simulink library "adrc"  (R2021a)
settings: Solver=VariableStepAuto  StartTime=0.0  StopTime=10.0  RelTol=1e-3
settings Model: Creator=onqi  LastModifiedBy=root

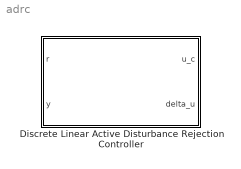
== system adrc ==
  Discrete Linear Active Disturbance Rejection Controller : Subsystem  Variant=on  VariantControl=Choice  mask(Linear Active Disturbance Rejection Control){order=1, b0=1, w_cl=1, k_eso=1, eso_init=[0;0], m_lim=[-inf, inf], r_lim=[-inf, inf], halfgain_ctrl=off, halfgain_obsv=off, inc_form=on, SampleTime=-1}
      mask prompts: order "First- or second-order ADRC"; b0 "Gain parameter b0"; w_cl "Desired closed-loop bandwidth w_cl [rad/s]"; k_eso "Relational observer bandwidth k_eso"; eso_init "Initial state of extended state observer"; m_lim "Magnitude limit of controller [lo, hi]"; r_lim "Rate limit of controller [lo, hi]"; halfgain_ctrl "Toggle half-gain tuning for controller"; halfgain_obsv "Toggle half-gain tuning for observer"; inc_form "Incremental form of ADRC"; SampleTime "Simulink:blkprm_prompts:AllBlksSampleTime"
      mask help:
      | Linear Active Disturbance Rejection Control block implementing the algorithms described in
      |
      | - Practical Active Disturbance Rejection Control: Bumpless Transfer, Rate Limitation and Incremental Algorithm, Gernot Herbst
      | - Half-Gain Tuning for Active Disturbance Rejection Control, Herbst et al.
      mask init:
      | ADRC_INC_FORM = inc_form;
      | 
      | if order == 1
      |     Ad = [[1, SampleTime];[0, 1]];
      |     Bd = [b0 * SampleTime; 0];
      |     Cd = [1, 0];
      |     Dd = 0;
      |     % Controller parameters for closed-loop dynamics
      |     t_settle = 4 / w_cl;
      |     sCL = -4 / t_settle;
      |     Kp = -2 * sCL;
      |     % Observer dynamics
      |     sESO = k_eso * sCL;
      |     zESO = exp(sESO * SampleTime);
      | 
      |     % Observer gains resulting in common-location observer poles
      |     L = [1 - zESO^2; (1 / SampleTime) * (1 - zESO)^2];
      | 
      |     % Controller gains
      |     w = [Kp / b0; 1 / b0];
      | 
      | elseif order == 2
      |     Ad = [[1, SampleTime, (SampleTime^2) / 2]; [0, 1, SampleTime]; [0, 0, 1]];
      |     Bd = [b0 * (SampleTime^2) / 2; b0 * SampleTime; 0];
      |     Cd = [1, 0, 0];
      |     Dd = 0;
      | 
      |     % Controller parameters for closed-loop dynamics
      |     t_settle = 6 / w_cl;
      |     sCL = -6 / t_settle;
      |     Kp = sCL^2;
      |     Kd = -2 * sCL;
      | 
      |     % Observer dynamics
      |     sESO = k_eso * sCL;
      |     zESO = exp(sESO * SampleTime);
      | 
      |     % Observer gains resulting in common-location observer poles
      |     L = [1 - (zESO)^3; (3 / (2 * SampleTime)) * (1 - zESO)^2 * (1 + zESO); 
      |         (1 / SampleTime^2) * (1 - zESO)^3];
      | 
      |     % Controller gains
      |     w = [Kp / b0; Kd / b0; 1 / b0];
      | end
      | 
      | if halfgain_obsv
      |     L = L/2;
      | end
      | 
      | if halfgain_ctrl
      |     w = w/2;
      | end
      | 
      | % One-step update equation implementing linear ESO
      | A_ESO = Ad - L * Cd * Ad;
      | B_ESO = Bd - L * Cd * Bd;
      | C_ESO = Cd;
      | 
      | L_ESO = L;
      settings: CopyFcn=set_param(gcbh,'LinkStatus','none');
      mask TypeOptions order: 1 | 2
      mask TypeOptions SampleTime: r/SampleTime
      mask DialogControl SampleTime Prompt: Sample time (-1 for inherited):
      mask Display:
      | disp('Discrete Linear\nADRC');
      | 
      | port_label('output', 1, 'u[k]', 'texmode', 'on');
      | port_label('input', 2, 'y[k-1]', 'texmode', 'on');
      | port_label('input', 1, 'r[k]', 'texmode', 'on');
      | 
      | if ADRC_INC_FORM == 1
      |     port_label('output', 2, '\Deltau', 'texmode', 'on');
      | end

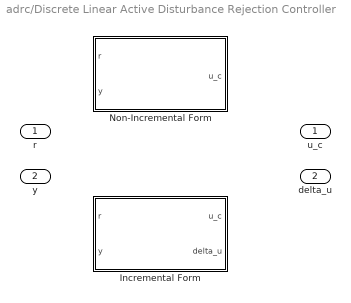
== system adrc/Discrete Linear Active Disturbance Rejection Controller ==
  r : Inport  SampleTime=SampleTime
  y : Inport  Port=2
  Incremental Form : Subsystem  VariantControl=inc_form == 1
  Non-Incremental Form : Subsystem  VariantControl=inc_form == 0
  u_c : Outport
  delta_u : Outport  Port=2

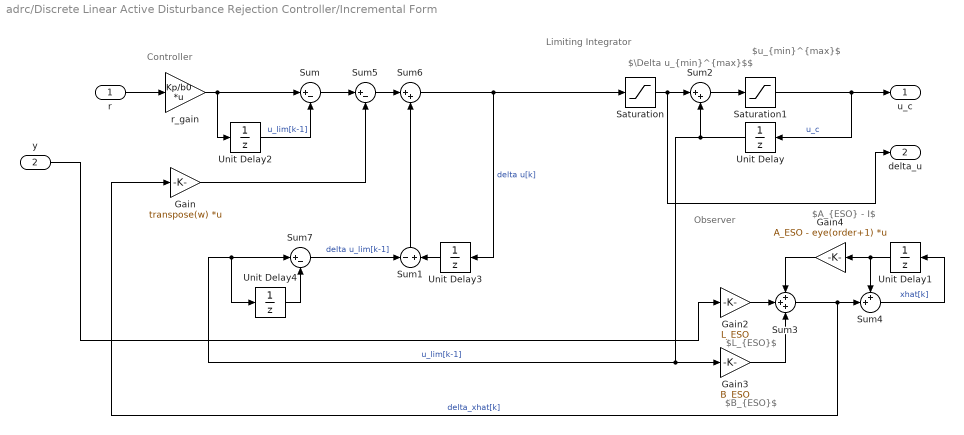
== system adrc/Discrete Linear Active Disturbance Rejection Controller/Incremental Form ==
  note: Controller
  note: $\Delta u_{min}^{max}$$
  note: $u_{min}^{max}$
  note: $L_{ESO}$
  note: $B_{ESO}$
  note: $A_{ESO} - I$
  note: Limiting
      | 	Integrator
  note: Observer
  r : Inport  SampleTime=SampleTime
  y : Inport  Port=2
  Gain : Gain  Gain=transpose(w)  Multiplication=Matrix(K*u) (u vector)
  Gain2 : Gain  Gain=L_ESO
  Gain3 : Gain  Gain=B_ESO
  Gain4 : Gain  Gain=A_ESO - eye(order+1)  Multiplication=Matrix(K*u) (u vector)
  Saturation : Saturate  UpperLimit=r_lim(2)  LowerLimit=r_lim(1)
  Saturation1 : Saturate  UpperLimit=m_lim(2)  LowerLimit=m_lim(1)
  Sum : Sum  Inputs=|+-
  Sum1 : Sum  Inputs=-+
  Sum2 : Sum  Inputs=|++
  Sum3 : Sum  Inputs=+++
  Sum4 : Sum  Inputs=++|
  Sum5 : Sum  Inputs=|+-
  Sum6 : Sum  Inputs=|++
  Sum7 : Sum  Inputs=|+-
  Unit Delay{,1..4} (5 alike) : UnitDelay  SampleTime=-1  HasFrameUpgradeWarning=on
  r_gain : Gain  Gain=Kp/b0  Multiplication=Matrix(K*u) (u vector)
  u_c : Outport
  delta_u : Outport  Port=2
  wires:
  Unit Delay1/1 -> Sum4/1, Gain4/1
  Sum2/1 -> Saturation1/1
  Gain4/1 -> Sum3/1
  Gain3/1 -> Sum3/3
  y/1 -> Gain2/1
  Sum6/1 -> Unit Delay3/1, Saturation/1  "delta u[k]"
  Saturation1/1 -> u_c/1, Unit Delay/1  "u_c"
  Unit Delay/1 -> Gain3/1, Unit Delay4/1, Sum7/1, Sum2/2  "u_lim[k-1]"
  Saturation/1 -> delta_u/1, Sum2/1
  r_gain/1 -> Unit Delay2/1, Sum/1
  r/1 -> r_gain/1
  Gain2/1 -> Sum3/2
  Sum4/1 -> Unit Delay1/1  "xhat[k]"
  Sum3/1 -> Gain/1, Sum4/2  "delta_xhat[k]"
  Sum/1 -> Sum5/1
  Sum5/1 -> Sum6/1
  Unit Delay2/1 -> Sum/2  "u_lim[k-1]"
  Gain/1 -> Sum5/2
  Unit Delay3/1 -> Sum1/2
  Sum1/1 -> Sum6/2
  Sum7/1 -> Sum1/1  "delta u_lim[k-1]"
  Unit Delay4/1 -> Sum7/2

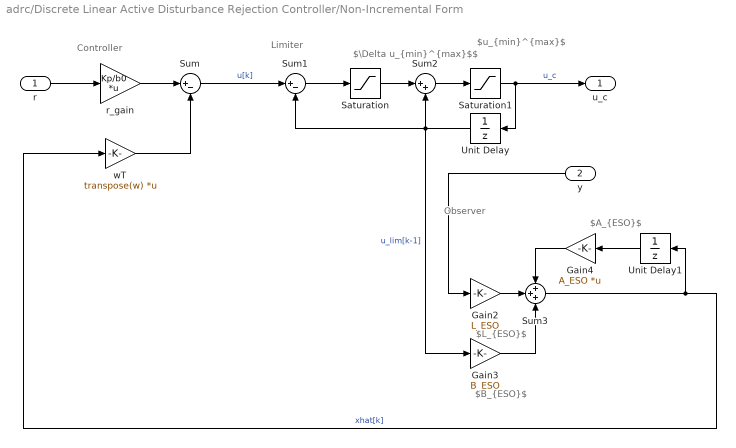
== system adrc/Discrete Linear Active Disturbance Rejection Controller/Non-Incremental Form ==
  note: Controller
  note: $\Delta u_{min}^{max}$$
  note: $u_{min}^{max}$
  note: $L_{ESO}$
  note: $B_{ESO}$
  note: $A_{ESO}$
  note: Limiter
  note: Observer
  r : Inport  SampleTime=SampleTime
  y : Inport  Port=2
  Gain2 : Gain  Gain=L_ESO
  Gain3 : Gain  Gain=B_ESO
  Gain4 : Gain  Gain=A_ESO  Multiplication=Matrix(K*u) (u vector)
  Saturation : Saturate  UpperLimit=r_lim(2)  LowerLimit=r_lim(1)
  Saturation1 : Saturate  UpperLimit=m_lim(2)  LowerLimit=m_lim(1)
  Sum : Sum  Inputs=|+-
  Sum1 : Sum  Inputs=|+-
  Sum2 : Sum  Inputs=|++
  Sum3 : Sum  Inputs=+++
  Unit Delay : UnitDelay  SampleTime=-1  HasFrameUpgradeWarning=on
  Unit Delay1 : UnitDelay  SampleTime=-1  HasFrameUpgradeWarning=on
  r_gain : Gain  Gain=Kp/b0  Multiplication=Matrix(K*u) (u vector)
  wT : Gain  Gain=transpose(w)  Multiplication=Matrix(K*u) (u vector)
  u_c : Outport
  wires:
  Unit Delay1/1 -> Gain4/1
  wT/1 -> Sum/2
  Sum2/1 -> Saturation1/1
  Gain4/1 -> Sum3/1
  Gain3/1 -> Sum3/3
  y/1 -> Gain2/1
  Sum1/1 -> Saturation/1
  Saturation1/1 -> u_c/1, Unit Delay/1  "u_c"
  Unit Delay/1 -> Gain3/1, Sum2/2, Sum1/2  "u_lim[k-1]"
  Saturation/1 -> Sum2/1
  r_gain/1 -> Sum/1
  r/1 -> r_gain/1
  Sum/1 -> Sum1/1  "u[k]"
  Sum3/1 -> wT/1, Unit Delay1/1  "xhat[k]"
  Gain2/1 -> Sum3/2
